simulink model "RSP"  (R2023a)
settings: Solver=FixedStepDiscrete  StartTime=0.0  StopTime=1.1*pri*N_observation  FixedStep=1.220703125E-8  RelTol=1e-3  EnableMultiTasking=on
model workspace (MAT data in the model file):
  Lambda : Simulink.Parameter (value not decoded)
  N_observation : Simulink.Parameter (value not decoded)
  N_sample : Simulink.Parameter (value not decoded)
  T_sampling : Simulink.Parameter (value not decoded)
  T_symbol : Simulink.Parameter (value not decoded)
  pri : Simulink.Parameter (value not decoded)
  symbol_delay : Simulink.Parameter (value not decoded)
symbols that are objects in the model workspace (value not decoded): Lambda, N_observation, N_sample, symbol_delay, T_sampling
libraries: hdlsllib x4, dsphdlxfrm2 x1
(part 15 of 49)

== matlab function RSP/Velocity Processor/Doppler Processing/Doppler Processor/Doppler Calculation ==
  data: u input; f output
function f  = fcn(u)
%#codegen

N = uint16(length(u));
max = fi(0,1,32,32);
idx_max = uint16(0);

for i=1:N/2
    if(u(i) > max )
        max = u(i);
        idx_max = i;
    end
end

f = fi(idx_max * 5000 / (N),0,32,5);
